simulink model "mtask4"  (R2019b)
settings: Solver=VariableStepAuto  StartTime=0.0  StopTime=10.0  RelTol=1e-3
undefined symbols (not defined in the file): k
settings Model: Creator=Jesus  LastModifiedBy=Jesus

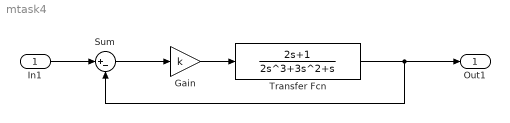
== system mtask4 ==
  In1 : Inport
  Gain : Gain  Gain=k
  Sum : Sum  Inputs=|+-
  Transfer Fcn : TransferFcn  Numerator=[2 1]  Denominator=[2 3 1 0]
  Out1 : Outport
  wires:
  In1/1 -> Sum/1
  Sum/1 -> Gain/1
  Gain/1 -> Transfer Fcn/1
  Transfer Fcn/1 -> Sum/2, Out1/1
